simulink model "example_9_2"  (R2023b)
settings: Solver=FixedStepAuto  StartTime=0.0  StopTime=20  FixedStep=0.01  RelTol=1e-6
libraries: commanapbnd3 x4
settings Model: Creator=wangh  LastModifiedBy=wangh

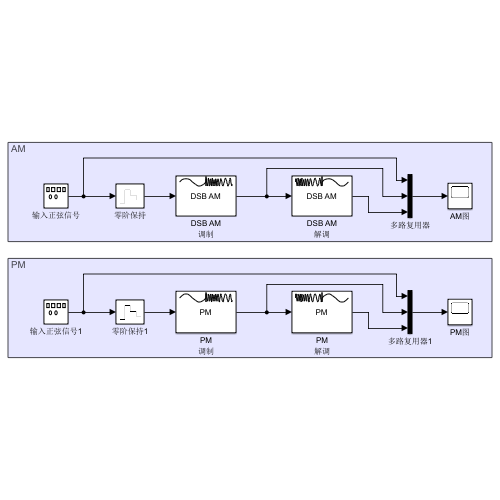
[thumbnail: Simulink's stored preview of the top-level diagram]
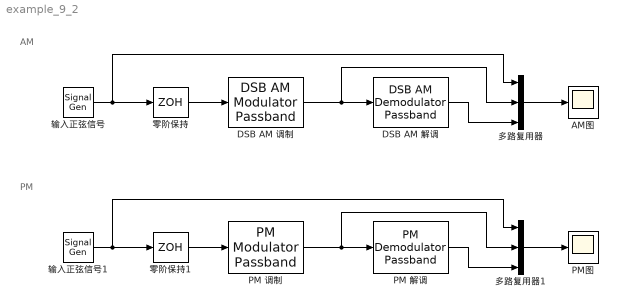
== system example_9_2 ==
  note: AM
  note: PM
  AM图 : Scope
  DSB AM 解调 : commanapbnd3/DSB AM Demodulator Passband  Fc=5  Ph=0  method=Butterworth  n=8  cf=2  Rp=0.1  Rs=50  Offset=0
  DSB AM 调制 : commanapbnd3/DSB AM Modulator Passband  Fc=5  Ph=0  Offset=0
  PM 解调 : commanapbnd3/PM Demodulator Passband  Fc=5  Ph=0  Kc=pi/2  Ho=8
  PM 调制 : commanapbnd3/PM Modulator Passband  Fc=5  Ph=0  Kc=pi/2
  PM图 : Scope
  多路复用器 : Mux  Inputs=3
  多路复用器1 : Mux  Inputs=3
  输入正弦信号 : SignalGenerator  Frequency=0.1
  输入正弦信号1 : SignalGenerator  Frequency=0.1
  零阶保持 : ZeroOrderHold  SampleTime=-1
  零阶保持1 : ZeroOrderHold  SampleTime=-1
  wires:
  DSB AM 调制/1 -> 多路复用器/2, DSB AM 解调/1
  输入正弦信号/1 -> 多路复用器/1, 零阶保持/1
  零阶保持/1 -> DSB AM 调制/1
  多路复用器/1 -> AM图/1
  DSB AM 解调/1 -> 多路复用器/3
  PM 解调/1 -> 多路复用器1/3
  多路复用器1/1 -> PM图/1
  零阶保持1/1 -> PM 调制/1
  输入正弦信号1/1 -> 零阶保持1/1, 多路复用器1/1
  PM 调制/1 -> PM 解调/1, 多路复用器1/2
